simulink model "MBDMotorSystemUpd2TrqReduce95"  (R2023a)
settings: Solver=VariableStepAuto  StartTime=0.0  StopTime=0.5  RelTol=1e-3
undefined symbols (not defined in the file): CntFdqDcpMap, CntLdqDMap, CntTrqReqMap, DiscIntNeverNeededParam, Izc, Izr, MaxLmtTrq, MdlFluxMap, MdlTrqMap, Pos0
libraries: simulink x30, simulink_extras x6
(part 3 of 4)

== system MBDMotorSystemUpd2TrqReduce95/PM Controller/PM Feedback Controller/dqAxis Limitation ==
  Lmt : Inport
  Fb : Inport  Port=2
  Complex to Magnitude-Angle : ComplexToMagnitudeAngle
  Complex to Real-Imag : ComplexToRealImag
  Constant : Constant  Value=0
  Demux : Demux  Outputs=2
  Fig VltStt1 : Scope  NumInputPorts=3
  Magnitude-Angle to Complex : MagnitudeAngleToComplex
  Mux : Mux  Inputs=2
  Real-Imag to Complex : RealImagToComplex
  Saturation Dynamic : simulink/Discontinuities/Saturation Dynamic  OutMin=[]  OutMax=[]  OutDataTypeStr=Inherit: Same as second input  OutDataType=fixdt(1, 16)  OutScaling=2^-10  DoSatur=off
  Sum2 : Sum  Inputs=-+|
  Val : Outport
  Delta : Outport  Port=2
  zVal : Outport  Port=3
  wires:
  Sum2/1 -> Delta/1
  Mux/1 -> Sum2/1, Val/1
  Demux/2 -> Real-Imag to Complex/2
  Demux/1 -> Real-Imag to Complex/1
  Constant/1 -> Saturation Dynamic/3
  Complex to Real-Imag/2 -> Mux/2
  Complex to Real-Imag/1 -> Mux/1
  Complex to Magnitude-Angle/2 -> Magnitude-Angle to Complex/2
  Saturation Dynamic/1 -> Fig VltStt1/2, Magnitude-Angle to Complex/1, zVal/1
  Fb/1 -> Demux/1, Sum2/2
  Complex to Magnitude-Angle/1 -> Fig VltStt1/1, Saturation Dynamic/2
  Lmt/1 -> Fig VltStt1/3, Saturation Dynamic/1
  Magnitude-Angle to Complex/1 -> Complex to Real-Imag/1
  Real-Imag to Complex/1 -> Complex to Magnitude-Angle/1

== system MBDMotorSystemUpd2TrqReduce95/PM Controller/PWM Timer/Base Modulator ==
  Fc : Inport
  Compare To Constant : simulink/Logic and Bit Operations/Compare To Constant  relop=<=  const=-1  OutDataTypeStr=boolean
  Compare To Constant1 : simulink/Logic and Bit Operations/Compare To Constant  relop=>=  const=1  OutDataTypeStr=boolean
  Data Type Conversion : DataTypeConversion  SaturateOnIntegerOverflow=off  RndMeth=Floor
  Fcn : Fcn  Expr=2*u(1)-1
  Gain : Gain  Gain=4
  Integrator : Integrator  InitialCondition=-1
  Math Function : Math  Operator=reciprocal  SignedPower=on
  Product : Product
  S-R Flip-Flop : simulink_extras/Flip Flops/S-R Flip-Flop  initial_condition=0
  Terminator : Terminator
  sampler : Subsystem  TreatAsAtomicUnit=on  mask{lTypTrigger=1: 山}
      mask prompts: lTypTrigger "更新トリガ"
      mask TypeOptions lTypTrigger: 0: 両方 | 1: 山 | 2: 谷
      mask Callback lTypTrigger:
      | if contains(get_param(gcbh,'lTypTrigger'),'山')
      |     set_param(getSimulinkBlockHandle([gcb,'/Trigger']),'TriggerType','rising')
      | elseif contains(get_param(gcbh,'lTypTrigger'),'谷')
      |     set_param(getSimulinkBlockHandle([gcb,'/Trigger']),'TriggerType','falling')
      | else
      |     set_param(getSimulinkBlockHandle([gcb,'/Trigger']),'TriggerType','either')
      | end
  "Trigger " : Outport
  Carrier : Outport  Port=2
  Tc : Outport  Port=3
  wires:
  sampler/1(Out1) -> Gain/1, Math Function/1
  Fc/1 -> sampler/1(In1)
  Gain/1 -> Product/2
  S-R Flip-Flop/2 -> Terminator/1
  Data Type Conversion/1 -> Fcn/1, "Trigger "/1
  Product/1 -> Integrator/1
  Compare To Constant1/1 -> S-R Flip-Flop/2
  Compare To Constant/1 -> S-R Flip-Flop/1
  S-R Flip-Flop/1 -> Data Type Conversion/1
  Fcn/1 -> Product/1, sampler/Trigger
  Integrator/1 -> Compare To Constant/1, Compare To Constant1/1, Carrier/1
  Math Function/1 -> Tc/1

== system MBDMotorSystemUpd2TrqReduce95/PM Controller/PWM Timer/DeadTime Correction ==
  Tdcs : Inport
  Iuvw : Inport  Port=2
  Abs : Abs  SaturateOnIntegerOverflow=off
  Constant : Constant  Value=0
  Constant1 : Constant  Value=[0 -vThr vThr]
  Constant2 : Constant  Value=0
  Constant5 : Constant  Value=vThr
  Constant7 : Constant
  Constant8 : Constant  Value=2
  Demux : Demux  Outputs=2
  Demux1 : Demux  Outputs=3
  Detect Change : simulink/Logic and Bit Operations/Detect Change  vinit=0  OutDataTypeStr=boolean
  Gain : Gain  Gain=kCrctTd
  Gain1 : Gain  Gain=0.5
  Logical Operator : Logic  Operator=NOR  AllPortsSameDT=off  OutDataTypeStr=boolean
  Multiport Switch : MultiPortSwitch  DataPortOrder=Zero-based contiguous  zeroidx=on  SaturateOnIntegerOverflow=off  InputSameDT=off
  Multiport Switch1 : MultiPortSwitch  DataPortOrder=Zero-based contiguous  zeroidx=on  SaturateOnIntegerOverflow=off  InputSameDT=off
  Relational Operator : RelationalOperator  Operator=>  OutDataTypeStr=boolean  RndMeth=Simplest  InputSameDT=off
  Relational Operator1 : RelationalOperator  Operator=>  OutDataTypeStr=boolean  RndMeth=Simplest  InputSameDT=off
  Switch : Switch  Criteria=u2 > Threshold  SaturateOnIntegerOverflow=off  InputSameDT=off
  Switch3 : Switch  Criteria=u2 > Threshold  SaturateOnIntegerOverflow=off  InputSameDT=off
  Unit Delay : UnitDelay  SampleTime=-1  HasFrameUpgradeWarning=on
  Tdc : Outport
  wires:
  Constant5/1 -> Gain1/1
  Gain1/1 -> Relational Operator/2
  Gain/1 -> Tdc/1
  Constant2/1 -> Multiport Switch/2
  Demux/2 -> Multiport Switch/4
  Demux/1 -> Multiport Switch/3
  Constant1/1 -> Demux1/1
  Demux1/3 -> Multiport Switch1/4
  Demux1/2 -> Multiport Switch1/3
  Demux1/1 -> Multiport Switch1/2
  Constant8/1 -> Switch3/3
  Multiport Switch1/1 -> Unit Delay/1
  Tdcs/1 -> Demux/1
  Switch/1 -> Multiport Switch/1, Multiport Switch1/1
  Multiport Switch/1 -> Gain/1
  Constant7/1 -> Switch3/1
  Relational Operator1/1 -> Switch3/2
  Constant/1 -> Switch/1
  Relational Operator/1 -> Logical Operator/2
  Detect Change/1 -> Logical Operator/1
  Abs/1 -> Relational Operator/1, Detect Change/1
  Iuvw/1 -> Abs/1, Relational Operator1/1
  Switch3/1 -> Switch/3
  Logical Operator/1 -> Switch/2
  Unit Delay/1 -> Relational Operator1/2

== system MBDMotorSystemUpd2TrqReduce95/PM Controller/PWM Timer/PWM Sampler ==
  v : Inport
  Trigger : TriggerPort  VariantControl=Variant
  s : Outport  InitialOutput=[0 0 0]
  wires:
  v/1 -> s/1

== system MBDMotorSystemUpd2TrqReduce95/PM Controller/PWM Timer/Signal Offset ==
  puvw : Inport
  Constant1 : Constant  Value=2
  Constant2 : Constant  Value=0
  Constant3 : Constant  Value=-2
  Demux : Demux  Outputs=3
  Mux : Mux  Inputs=3
  Sum2 : Sum  Inputs=++|
  Sum3 : Sum  Inputs=++|
  Sum4 : Sum  Inputs=++|
  Pwm SigOuts : Outport
  wires:
  Demux/1 -> Sum2/1
  Demux/2 -> Sum3/1
  Demux/3 -> Sum4/1
  puvw/1 -> Demux/1
  Constant1/1 -> Sum2/2
  Mux/1 -> Pwm SigOuts/1
  Constant2/1 -> Sum3/2
  Sum4/1 -> Mux/3
  Constant3/1 -> Sum4/2
  Sum2/1 -> Mux/1
  Sum3/1 -> Mux/2

== system MBDMotorSystemUpd2TrqReduce95/PM Controller/Resolver Settings/Resolver Error ==
  note: 代数ループ回避
      | 誤差なので問題無と
  note: 乱数は，乱数発生器 rng での初期化が場合により必要です．
  note: 必要に応じて，追加・削除・変更して下さい．
  note: 各位置毎にテーブルでエラー設定
      | その間を線形補間
  Pos Rez. [deg.] : Inport
  Fail : Inport  Port=2
  Constant : Constant  Value=0.5
  Constant1 : Constant  Value=0
  Error Mode : Constant  Value=0
  Gain : Gain  Gain=10
  Gain1 : Gain  Gain=20
  Gain2 : Gain  Gain=2
  Manual Switch : ManualSwitch  CurrentSetting=0
  Memory : Memory  Commented=through
  Multiport Switch : MultiPortSwitch  DataPortOrder=Zero-based contiguous  Inputs=4  DataPortForDefault=Additional data port  DiagnosticForDefault=Warning  zeroidx=on  SaturateOnIntegerOverflow=off  InputSameDT=off
  Ramdom Error : Lookup_n-D  NumberOfTableDimensions=1  BreakpointsForDimension1=0:360  Table=rand(1,361)  InternalRulePriority=Speed  RndMeth=Simplest
  Sin Error : Lookup_n-D  NumberOfTableDimensions=1  BreakpointsForDimension1=0:360  Table=sind(0:360)  InternalRulePriority=Speed  RndMeth=Simplest
  Sum : Sum  Inputs=|+-
  Table Error : Lookup_n-D  NumberOfTableDimensions=1  BreakpointsForDimension1=0:30:360  BeginIndexSearchUsingPreviousIndexResult=on  Table=[10 30 -50 80 -10 50 -100 20 -50 70 -30 -80 10]  InternalRulePriority=Speed  RndMeth=Simplest
  Err. [deg.] : Outport
  wires:
  Pos Rez. [deg.]/1 -> Table Error/1, Ramdom Error/1, Sin Error/1
  Ramdom Error/1 -> Sum/1
  Sum/1 -> Gain2/1
  Constant/1 -> Sum/2
  Sin Error/1 -> Gain1/1
  Multiport Switch/1 -> Memory/1
  Manual Switch/1 -> Multiport Switch/6, Multiport Switch/1
  Gain2/1 -> Gain/1
  Memory/1 -> Err. [deg.]/1
  Gain1/1 -> Multiport Switch/5
  Gain/1 -> Multiport Switch/4
  Table Error/1 -> Multiport Switch/3
  Error Mode/1 -> Manual Switch/1
  Fail/1 -> Manual Switch/2
  Constant1/1 -> Multiport Switch/2

== system MBDMotorSystemUpd2TrqReduce95/PM Controller/Resolver Settings/Resolver Fail ==
  Pos. Mech. [deg.] : Inport
  Fail Speed [rpm] : Inport  Port=2
  Fail : Inport  Port=3
  Compare To Constant : simulink/Logic and Bit Operations/Compare To Constant  relop=<  const=0.5  OutDataTypeStr=boolean
  Gain1 : Gain  Gain=6
  Integrator1 : Integrator  ExternalReset=level  InitialConditionSource=external  InitialCondition=Pos0  WrapState=on  WrappedStateUpperValue=360  WrappedStateLowerValue=0
  NOT : Logic  Operator=NOT  IconShape=distinctive  AllPortsSameDT=off  OutDataTypeStr=boolean
  Switch : Switch  Criteria=u2 > Threshold  SaturateOnIntegerOverflow=off  InputSameDT=off
  Pos. Mech. [deg] : Outport
  wires:
  NOT/1 -> Switch/2
  Fail Speed [rpm]/1 -> Gain1/1
  Gain1/1 -> Integrator1/1
  Pos. Mech. [deg.]/1 -> Switch/3, Integrator1/3
  Compare To Constant/1 -> Integrator1/2, NOT/1
  Fail/1 -> Compare To Constant/1
  Integrator1/1 -> Switch/1
  Switch/1 -> Pos. Mech. [deg]/1

== system MBDMotorSystemUpd2TrqReduce95/Power Source/Power Source Cable Cs/Cable LR ==
  note: Inner Status
  Vin : Inport
  Vo : Inport  Port=2
  Ib0 : Inport  Port=3
  Bus Creator2 : BusCreator  Inputs=3
  Bus Creator3 : BusCreator  Inputs=3
  Constant1 : Constant  Value=0
  Constant2 : Constant  Value=0
  Divide2 : Product  Inputs=*/
  Integrator1 : Integrator  InitialConditionSource=external  LowerSaturationLimit=0
  IsRc : VariantSource  VariantControlMode=label  LabelModeActiveChoice=Off  ShowConditionOnBlock=on
  Product1 : Product
  Sum2 : Sum  Inputs=+-
  Sum6 : Sum  Inputs=+-
  vLc : Constant  Value=1e-06
  vRc : Constant  Value=0.001
  Ib : Outport
  Stt : Outport  Port=2
  wires:
  vLc/1 -> Divide2/2
  Divide2/1 -> Integrator1/1
  Integrator1/1 -> [Ib], Product1/1, Ib/1
  Vin/1 -> Sum6/1
  Vo/1 -> [Vo], Sum6/2
  vRc/1 -> Product1/2
  Ib0/1 -> Integrator1/2
  Sum6/1 -> [Vcl], Sum2/1
  Constant2/1 -> IsRc/1
  Product1/1 -> IsRc/2
  Sum2/1 -> Divide2/1
  IsRc/1 -> [Vcr], Sum2/2
  [Vcr] -> Bus Creator3/3  "Vcr"
  [Ib] -> Bus Creator2/2  "Ib"
  Constant1/1 -> Bus Creator3/2  "Icc"
  [Vcl] -> Bus Creator3/1  "Vcl"
  Bus Creator3/1 -> Bus Creator2/3  "InStt"
  Bus Creator2/1 -> Stt/1  "CblStt"
  [Vo] -> Bus Creator2/1  "Vo"

== system MBDMotorSystemUpd2TrqReduce95/Power Source/Power Source Cable Cs/Cable LRC ==
  note: Inner Status
  Vin : Inport
  Io : Inport  Port=2
  V0 : Inport  Port=3
  Bus Creator : BusCreator  Inputs=3
  Bus Creator1 : BusCreator  Inputs=3
  Constant4 : Constant  Value=0
  Divide1 : Product  Inputs=*/
  Divide2 : Product  Inputs=*/
  Integrator : Integrator  InitialConditionSource=external  LimitOutput=on  LowerSaturationLimit=0
  Integrator1 : Integrator  LowerSaturationLimit=0
  IsRc : VariantSource  VariantControlMode=label  LabelModeActiveChoice=Off  ShowConditionOnBlock=on
  Product1 : Product
  Sum1 : Sum  Inputs=+-
  Sum2 : Sum  Inputs=+-
  Sum6 : Sum  Inputs=+-
  vCc : Constant  Value=1e-06
  vLc : Constant  Value=1e-06
  vRc : Constant  Value=0.001
  Vo : Outport
  Ib : Outport  Port=2
  Stt : Outport  Port=3
  wires:
  IsRc/1 -> Sum2/2, [Vcr]
  vRc/1 -> Product1/2
  Constant4/1 -> IsRc/1
  Bus Creator1/1 -> Bus Creator/3  "InStt"
  [Vcr] -> Bus Creator1/3  "Vcr"
  [Icc] -> Bus Creator1/2  "Icc"
  [Vcl] -> Bus Creator1/1  "Vcl"
  [Ib] -> Bus Creator/2  "Ib"
  [Vo] -> Bus Creator/1  "Vo"
  Bus Creator/1 -> Stt/1  "CblStt"
  Io/1 -> Sum1/2
  Integrator/1 -> [Vo], Sum6/2, Vo/1
  Divide1/1 -> Integrator/1
  vCc/1 -> Divide1/2
  Sum1/1 -> Divide1/1, [Icc]
  Product1/1 -> IsRc/2
  Sum6/1 -> Sum2/1
  Vin/1 -> Sum6/1
  Integrator1/1 -> [Ib], Product1/1, Sum1/1, Ib/1
  Divide2/1 -> Integrator1/1
  Sum2/1 -> Divide2/1, [Vcl]
  vLc/1 -> Divide2/2
  V0/1 -> Integrator/2

== system MBDMotorSystemUpd2TrqReduce95/Power Source/Power Source Cable Cs/Cs No ESL ==
  note: Inner Status
  I Load : Inport
  Ib : Inport  Port=2
  V0in : Inport  Port=3
  Bus Creator2 : BusCreator  Inputs=3
  Bus Creator3 : BusCreator  Inputs=3
  Constant2 : Constant  Value=0
  Divide : Product  Inputs=*/
  Divide1 : Product  Inputs=*/
  Integrator : Integrator  InitialConditionSource=external  LimitOutput=on  LowerSaturationLimit=0
  IsESR : VariantSource  VariantControlMode=label  LabelModeActiveChoice=Off  ShowConditionOnBlock=on
  IsESRini : VariantSource  VariantControlMode=label  LabelModeActiveChoice=Off  ShowConditionOnBlock=on
  Product : Product
  Sum1 : Sum  Inputs=+-
  Sum2 : Sum
  Sum3 : Sum  Inputs=+-
  Sum4 : Sum  Inputs=-+
  isIR : VariantSource  VariantControlMode=label  LabelModeActiveChoice=Off  ShowConditionOnBlock=on
  vCsU : Constant  Value=Cs
  vESR : Constant  Value=ESR
  vIR : Constant  Value=IR
  Vdc : Outport
  Stt : Outport  Port=2
  wires:
  Sum4/1 -> IsESRini/1
  V0in/1 -> Sum4/2, IsESRini/2
  Integrator/1 -> [Vcs], Sum2/2, Divide1/1
  Divide/1 -> Integrator/1
  vESR/1 -> Product/1
  vCsU/1 -> Divide/2
  I Load/1 -> Sum1/2
  Ib/1 -> Sum1/1
  [Vesr] -> Sum4/1
  isIR/1 -> [Is], Divide/1
  Divide1/1 -> [Iir], Sum3/2
  Sum3/1 -> isIR/2
  Sum1/1 -> Sum3/1, isIR/1, Product/2
  vIR/1 -> Divide1/2
  IsESR/1 -> [Vesr], Sum2/1
  Sum2/1 -> [Vdc], Vdc/1
  Constant2/1 -> IsESR/2
  Product/1 -> IsESR/1
  [Vdc] -> Bus Creator2/1  "Vin"
  [Iir] -> Bus Creator3/3  "Iir"
  [Vcs] -> Bus Creator3/1  "Vcs"
  Bus Creator2/1 -> Stt/1  "CsStt"
  [Vesr] -> Bus Creator3/2  "Ver"
  [Is] -> Bus Creator2/2  "Is"
  Bus Creator3/1 -> Bus Creator2/3  "InStt"
  IsESRini/1 -> Integrator/2

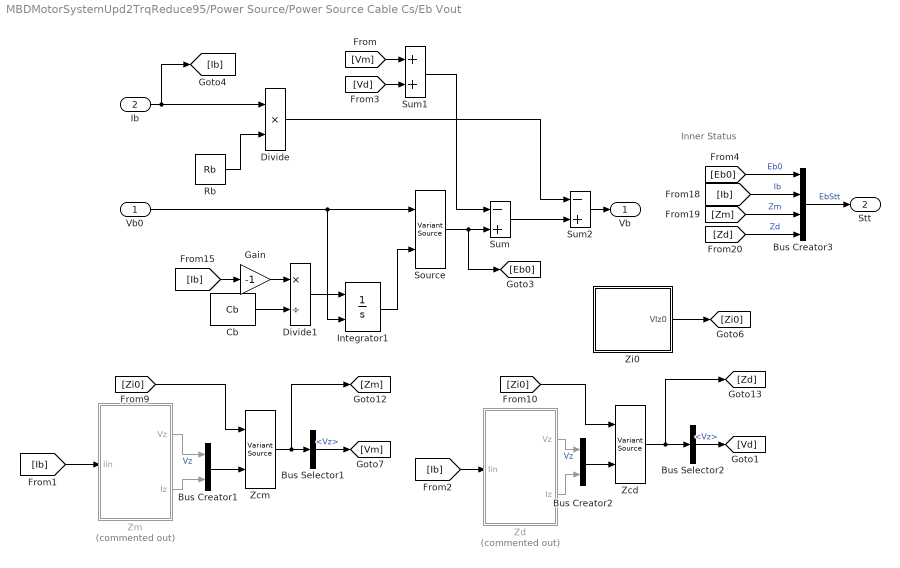
== system MBDMotorSystemUpd2TrqReduce95/Power Source/Power Source Cable Cs/Eb Vout ==
  note: Inner Status
  Vb0 : Inport
  Ib : Inport  Port=2
  Bus Creator1 : BusCreator  Inputs=2
  Bus Creator2 : BusCreator  Inputs=2
  Bus Creator3 : BusCreator  Inputs=4
  Bus Selector1 : BusSelector  OutputSignals=Vz
  Bus Selector2 : BusSelector  OutputSignals=Vz
  Cb : Constant  Value=Cb
  Divide : Product
  Divide1 : Product  Inputs=*/
  Gain : Gain  Gain=-1
  Integrator1 : Integrator  InitialConditionSource=external  LimitOutput=on  LowerSaturationLimit=0
  Rb : Constant  Value=Rb
  Source : VariantSource  VariantControlMode=label  LabelModeActiveChoice=PS  ShowConditionOnBlock=on
  Sum : Sum  Inputs=-+
  Sum1 : Sum
  Sum2 : Sum  Inputs=-+
  Zcd : VariantSource  VariantControlMode=label  LabelModeActiveChoice=Off  ShowConditionOnBlock=on
  Zcm : VariantSource  VariantControlMode=label  LabelModeActiveChoice=Off  ShowConditionOnBlock=on
  Zd : Subsystem  Commented=on  mask{Cz=Cd, Rz=Rd}
      mask prompts: Cz "内部インピーダンス容量 [C]"; Rz "内部インピーダンス抵抗 [Ω]"
      mask DialogControl ParameterGroupVar Prompt: パラメーター
  Zi0 : Subsystem
  Zm : Subsystem  Commented=on  mask{Cz=Cm, Rz=Rm}
      mask prompts: Cz "内部インピーダンス容量 [C]"; Rz "内部インピーダンス抵抗 [Ω]"
      mask DialogControl ParameterGroupVar Prompt: パラメーター
  Vb : Outport
  Stt : Outport  Port=2
  wires:
  Bus Creator3/1 -> Stt/1  "EbStt"
  [Zm] -> Bus Creator3/3  "Zm"
  [Eb0] -> Bus Creator3/1  "Eb0"
  [Ib] -> Bus Creator3/2  "Ib"
  [Zd] -> Bus Creator3/4  "Zd"
  [Zi0] -> Zcd/1
  Zcd/1 -> Bus Selector2/1, [Zd]
  Bus Selector2/1 -> [Vd]  "<Vz>"
  Zd/1(Vz) -> Bus Creator2/1  "Vz"
  Bus Creator2/1 -> Zcd/2
  Zd/2(Iz) -> Bus Creator2/2
  Zcm/1 -> Bus Selector1/1, [Zm]
  [Zi0] -> Zcm/1
  Bus Creator1/1 -> Zcm/2
  Zm/1(Vz) -> Bus Creator1/1  "Vz"
  Zm/2(Iz) -> Bus Creator1/2
  Bus Selector1/1 -> [Vm]  "<Vz>"
  Zi0/1(VIz0) -> [Zi0]
  [Ib] -> Zm/1(Iin)
  [Ib] -> Gain/1
  Rb/1 -> Divide/2
  Ib/1 -> Divide/1, [Ib]
  Sum/1 -> Sum2/2
  Gain/1 -> Divide1/1
  Divide1/1 -> Integrator1/1
  Cb/1 -> Divide1/2
  Vb0/1 -> Integrator1/2, Source/1
  Integrator1/1 -> Source/2
  Source/1 -> [Eb0], Sum/2
  [Vm] -> Sum1/1
  [Vd] -> Sum1/2
  Sum1/1 -> Sum/1
  Sum2/1 -> Vb/1
  Divide/1 -> Sum2/1
  [Ib] -> Zd/1(Iin)

== system MBDMotorSystemUpd2TrqReduce95/Power Source/Power Source Cs/Cs No ESL ==
  note: Inner Status
  I Load : Inport
  Ib : Inport  Port=2
  V0in : Inport  Port=3
  Bus Creator2 : BusCreator  Inputs=3
  Bus Creator3 : BusCreator  Inputs=3
  Constant2 : Constant  Value=0
  Divide : Product  Inputs=*/
  Divide1 : Product  Inputs=*/
  Integrator : Integrator  InitialConditionSource=external  LimitOutput=on  LowerSaturationLimit=0
  IsESR : VariantSource  VariantControlMode=label  LabelModeActiveChoice=Off  ShowConditionOnBlock=on
  IsESRini : VariantSource  VariantControlMode=label  LabelModeActiveChoice=Off  ShowConditionOnBlock=on
  Product : Product
  Sum1 : Sum  Inputs=+-
  Sum2 : Sum
  Sum3 : Sum  Inputs=+-
  Sum4 : Sum  Inputs=-+
  isIR : VariantSource  VariantControlMode=label  LabelModeActiveChoice=Off  ShowConditionOnBlock=on
  vCsU : Constant  Value=Cs
  vESR : Constant  Value=ESR
  vIR : Constant  Value=IR
  Vdc : Outport
  Stt : Outport  Port=2
  wires:
  Sum4/1 -> IsESRini/1
  V0in/1 -> Sum4/2, IsESRini/2
  Integrator/1 -> [Vcs], Sum2/2, Divide1/1
  Divide/1 -> Integrator/1
  vESR/1 -> Product/1
  vCsU/1 -> Divide/2
  I Load/1 -> Sum1/2
  Ib/1 -> Sum1/1
  [Vesr] -> Sum4/1
  isIR/1 -> [Is], Divide/1
  Divide1/1 -> [Iir], Sum3/2
  Sum3/1 -> isIR/2
  Sum1/1 -> Sum3/1, isIR/1, Product/2
  vIR/1 -> Divide1/2
  IsESR/1 -> [Vesr], Sum2/1
  Sum2/1 -> [Vdc], Vdc/1
  Constant2/1 -> IsESR/2
  Product/1 -> IsESR/1
  [Vdc] -> Bus Creator2/1  "Vin"
  [Iir] -> Bus Creator3/3  "Iir"
  [Vcs] -> Bus Creator3/1  "Vcs"
  Bus Creator2/1 -> Stt/1  "CsStt"
  [Vesr] -> Bus Creator3/2  "Ver"
  [Is] -> Bus Creator2/2  "Is"
  Bus Creator3/1 -> Bus Creator2/3  "InStt"
  IsESRini/1 -> Integrator/2

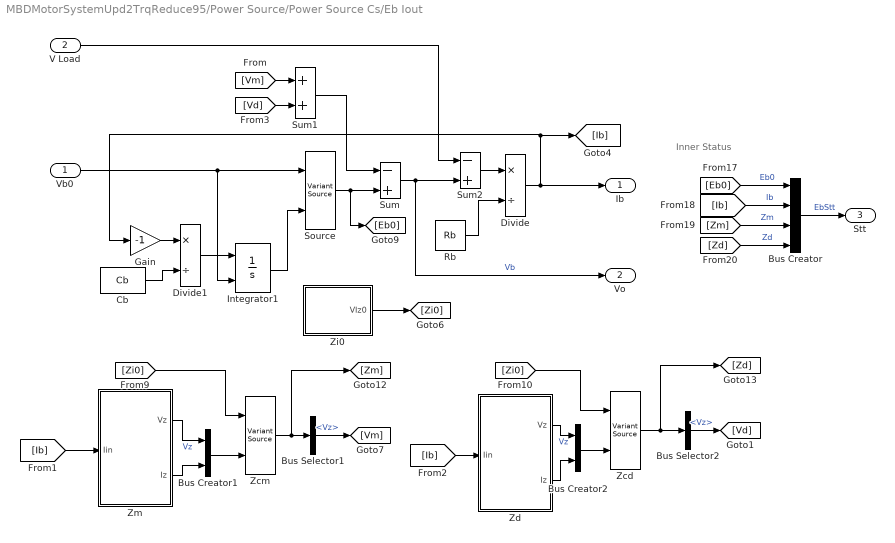
== system MBDMotorSystemUpd2TrqReduce95/Power Source/Power Source Cs/Eb Iout ==
  note: Inner Status
  Vb0 : Inport
  V Load : Inport  Port=2
  Bus Creator : BusCreator  Inputs=4
  Bus Creator1 : BusCreator  Inputs=2
  Bus Creator2 : BusCreator  Inputs=2
  Bus Selector1 : BusSelector  OutputSignals=Vz
  Bus Selector2 : BusSelector  OutputSignals=Vz
  Cb : Constant  Value=Cb
  Divide : Product  Inputs=*/
  Divide1 : Product  Inputs=*/
  Gain : Gain  Gain=-1
  Integrator1 : Integrator  InitialConditionSource=external
  Rb : Constant  Value=Rb
  Source : VariantSource  VariantControlMode=label  LabelModeActiveChoice=PS  ShowConditionOnBlock=on
  Sum : Sum  Inputs=-+
  Sum1 : Sum
  Sum2 : Sum  Inputs=-+
  Zcd : VariantSource  VariantControlMode=label  LabelModeActiveChoice=Off  ShowConditionOnBlock=on
  Zcm : VariantSource  VariantControlMode=label  LabelModeActiveChoice=Off  ShowConditionOnBlock=on
  Zd : Subsystem  mask{Cz=Cd, Rz=Rd}
      mask prompts: Cz "内部インピーダンス容量 [C]"; Rz "内部インピーダンス抵抗 [Ω]"
      mask DialogControl ParameterGroupVar Prompt: パラメーター
  Zi0 : Subsystem
  Zm : Subsystem  mask{Cz=Cm, Rz=Rm}
      mask prompts: Cz "内部インピーダンス容量 [C]"; Rz "内部インピーダンス抵抗 [Ω]"
      mask DialogControl ParameterGroupVar Prompt: パラメーター
  Ib : Outport
  Vo : Outport  Port=2
  Stt : Outport  Port=3
  wires:
  [Zi0] -> Zcm/1
  [Ib] -> Zd/1(Iin)
  [Ib] -> Zm/1(Iin)
  [Zi0] -> Zcd/1
  Zcm/1 -> Bus Selector1/1, [Zm]
  Zm/2(Iz) -> Bus Creator1/2
  Bus Selector1/1 -> [Vm]  "<Vz>"
  Zd/2(Iz) -> Bus Creator2/2
  Bus Creator2/1 -> Zcd/2
  Bus Selector2/1 -> [Vd]  "<Vz>"
  Bus Creator1/1 -> Zcm/2
  Zd/1(Vz) -> Bus Creator2/1  "Vz"
  Zcd/1 -> Bus Selector2/1, [Zd]
  Zm/1(Vz) -> Bus Creator1/1  "Vz"
  Bus Creator/1 -> Stt/1  "EbStt"
  [Zd] -> Bus Creator/4  "Zd"
  [Zm] -> Bus Creator/3  "Zm"
  [Ib] -> Bus Creator/2  "Ib"
  [Eb0] -> Bus Creator/1  "Eb0"
  Zi0/1(VIz0) -> [Zi0]
  V Load/1 -> Sum2/1
  Sum2/1 -> Divide/1
  Sum1/1 -> Sum/1
  [Vd] -> Sum1/2
  [Vm] -> Sum1/1
  Source/1 -> Sum/2, [Eb0]
  Integrator1/1 -> Source/2
  Vb0/1 -> Source/1, Integrator1/2
  Cb/1 -> Divide1/2
  Divide/1 -> Gain/1, [Ib], Ib/1
  Divide1/1 -> Integrator1/1
  Gain/1 -> Divide1/1
  Rb/1 -> Divide/2
  Sum/1 -> Vo/1, Sum2/2  "Vb"

== system MBDMotorSystemUpd2TrqReduce95/PM Controller/Modulator/Over Modulation/Ovr. Mod. ==
  PWM Mode : Inport
  Mr : Inport  Port=2
  Action Port : ActionPort  ActionPortLabel=if(u1 > 0)
  Gain : Gain  Gain=sqrt(2)/2
  Gain1 : Gain  Gain=sqrt(2)
  Merge : Merge  Inputs=3
  OvrMod. DPWM : Subsystem  TreatAsAtomicUnit=on
  OvrMod. SPWM : Subsystem  TreatAsAtomicUnit=on
  OvrMod. SVM : Subsystem  TreatAsAtomicUnit=on
  Switch Case : SwitchCase  CaseConditions={0, 1}
  Mr* : Outport
  wires:
  Switch Case/3 -> OvrMod. SPWM/Action
  OvrMod. SVM/1(Mr*) -> Merge/1
  Mr/1 -> Gain/1
  OvrMod. DPWM/1(Mr*) -> Merge/2
  Switch Case/2 -> OvrMod. DPWM/Action
  OvrMod. SPWM/1(Mr*) -> Merge/3
  PWM Mode/1 -> Switch Case/1
  Merge/1 -> Gain1/1
  Switch Case/1 -> OvrMod. SVM/Action
  Gain/1 -> OvrMod. SVM/1(Mr), OvrMod. DPWM/1(Mr), OvrMod. SPWM/1(Mr)
  Gain1/1 -> Mr*/1

== system MBDMotorSystemUpd2TrqReduce95/PM Controller/Modulator/Over Modulation/Through ==
  Mr : Inport
  Action Port : ActionPort  ActionPortLabel=else
  Mr* : Outport
  wires:
  Mr/1 -> Mr*/1

== system MBDMotorSystemUpd2TrqReduce95/PM Controller/Modulator/Vz Correction/DPWM ==
  VaReq : Inport
  MaxVa : Inport  Port=2
  Action Port : ActionPort  ActionPortLabel=case [ 1 ]:
  Abs : Abs  SaturateOnIntegerOverflow=off
  Abs1 : Abs  SaturateOnIntegerOverflow=off
  Demux3 : Demux  Outputs=3
  Demux4 : Demux  Outputs=3
  Gain : Gain  Gain=-1
  Max : MinMax  Function=max  Inputs=3  ZeroCross=off
  Max1 : MinMax  Inputs=3  ZeroCross=off
  Relational Operator3 : RelationalOperator  OutDataTypeStr=boolean  ZeroCross=off  RndMeth=Simplest  InputSameDT=off
  Sum : Sum  Inputs=-+
  Sum2 : Sum  Inputs=+-
  Switch : Switch  Criteria=u2 > Threshold  SaturateOnIntegerOverflow=off  InputSameDT=off
  Vz : Outport
  wires:
  Demux3/2 -> Max/2
  Max1/1 -> Sum/1, Abs1/1
  Demux4/3 -> Max1/3
  Demux4/2 -> Max1/2
  Demux3/3 -> Max/3
  Abs1/1 -> Relational Operator3/2
  Max/1 -> Sum2/2, Abs/1
  Abs/1 -> Relational Operator3/1
  Sum2/1 -> Switch/1
  Sum/1 -> Switch/3
  Relational Operator3/1 -> Switch/2
  VaReq/1 -> Demux3/1, Demux4/1
  Demux3/1 -> Max/1
  Demux4/1 -> Max1/1
  Switch/1 -> Vz/1
  MaxVa/1 -> [MaxVa]
  [MaxVa] -> Gain/1
  Gain/1 -> Sum/2
  [MaxVa] -> Sum2/1

== system MBDMotorSystemUpd2TrqReduce95/PM Controller/Modulator/Vz Correction/Nothing ==
  Action Port : ActionPort  ActionPortLabel=default:
  Constant : Constant  Value=0
  Vz : Outport
  wires:
  Constant/1 -> Vz/1

== system MBDMotorSystemUpd2TrqReduce95/PM Controller/Modulator/Vz Correction/SVM ==
  VaReq : Inport
  Action Port : ActionPort  ActionPortLabel=case [ 0 ]:
  Demux4 : Demux  Outputs=3
  Demux5 : Demux  Outputs=3
  Gain : Gain  Gain=-0.5
  Max : MinMax  Function=max  Inputs=3  ZeroCross=off
  Max1 : MinMax  Inputs=3  ZeroCross=off
  Mux : Mux  Inputs=2
  Sum of Elements : Sum  Inputs=+
  Vz : Outport
  wires:
  VaReq/1 -> Demux4/1, Demux5/1
  Sum of Elements/1 -> Gain/1
  Demux4/1 -> Max/1
  Demux4/3 -> Max/3
  Mux/1 -> Sum of Elements/1
  Gain/1 -> Vz/1
  Max1/1 -> Mux/2
  Demux5/1 -> Max1/1
  Demux5/3 -> Max1/3
  Max/1 -> Mux/1
  Demux5/2 -> Max1/2
  Demux4/2 -> Max/2

== system MBDMotorSystemUpd2TrqReduce95/PM Controller/PWM Timer/Base Modulator/sampler ==
  In1 : Inport
  Trigger : TriggerPort  VariantControl=Variant  InitialTriggerSignalState=zero
  Out1 : Outport
  wires:
  In1/1 -> Out1/1

== system MBDMotorSystemUpd2TrqReduce95/Power Source/Power Source Cable Cs/Eb Vout/Zd ==
  Iin : Inport
  Cz : Constant  Value=Cz
  Divide : Product  Inputs=*/
  Divide1 : Product  Inputs=*/
  Integrator : Integrator  InitialConditionSource=external
  Istt : BusCreator  Inputs=Izr,Izc
  Product : Product
  Rz : Constant  Value=Rz
  Sum : Sum  Inputs=-+
  Vz : Outport
  Iz : Outport  Port=2
  wires:
  Integrator/1 -> Divide1/1, Vz/1  "Vz"
  Istt/1 -> Iz/1  "Iz"
  Divide/1 -> Integrator/1
  Rz/1 -> Product/1, Divide1/2
  Iin/1 -> Sum/2, Product/2
  Sum/1 -> Istt/2, Divide/1  "Izc"
  Divide1/1 -> Istt/1, Sum/1  "Izr"
  Product/1 -> Integrator/2
  Cz/1 -> Divide/2

== system MBDMotorSystemUpd2TrqReduce95/Power Source/Power Source Cable Cs/Eb Vout/Zi0 ==
  Constant2 : Constant  Value=NaN
  Constant3 : Constant  Value=NaN
  Constant4 : Constant  Value=0
  Iz : BusCreator  Inputs=Izr,Izc
  VIz : BusCreator  Inputs=2
  VIz0 : Outport
  wires:
  Constant2/1 -> Iz/2  "Izc"
  Iz/1 -> VIz/2  "Iz"
  VIz/1 -> VIz0/1  "VIz"
  Constant3/1 -> Iz/1  "Izr"
  Constant4/1 -> VIz/1  "Vz"

== system MBDMotorSystemUpd2TrqReduce95/Power Source/Power Source Cable Cs/Eb Vout/Zm ==
  Iin : Inport
  Cz : Constant  Value=Cz
  Divide : Product  Inputs=*/
  Divide1 : Product  Inputs=*/
  Integrator : Integrator  InitialConditionSource=external
  Istt : BusCreator  Inputs=Izr,Izc
  Product : Product
  Rz : Constant  Value=Rz
  Sum : Sum  Inputs=-+
  Vz : Outport
  Iz : Outport  Port=2
  wires:
  Divide/1 -> Integrator/1
  Divide1/1 -> Istt/1, Sum/1  "Izr"
  Sum/1 -> Istt/2, Divide/1  "Izc"
  Cz/1 -> Divide/2
  Istt/1 -> Iz/1  "Iz"
  Product/1 -> Integrator/2
  Iin/1 -> Sum/2, Product/2
  Rz/1 -> Product/1, Divide1/2
  Integrator/1 -> Divide1/1, Vz/1  "Vz"

== system MBDMotorSystemUpd2TrqReduce95/Power Source/Power Source Cs/Eb Iout/Zd ==
  Iin : Inport
  Cz : Constant  Value=Cz
  Divide : Product  Inputs=*/
  Divide1 : Product  Inputs=*/
  Integrator : Integrator  InitialConditionSource=external
  Istt : BusCreator  Inputs=Izr,Izc
  Product : Product
  Rz : Constant  Value=Rz
  Sum : Sum  Inputs=-+
  Vz : Outport
  Iz : Outport  Port=2
  wires:
  Integrator/1 -> Divide1/1, Vz/1  "Vz"
  Istt/1 -> Iz/1  "Iz"
  Divide/1 -> Integrator/1
  Rz/1 -> Product/1, Divide1/2
  Iin/1 -> Sum/2, Product/2
  Sum/1 -> Istt/2, Divide/1  "Izc"
  Divide1/1 -> Istt/1, Sum/1  "Izr"
  Product/1 -> Integrator/2
  Cz/1 -> Divide/2

== system MBDMotorSystemUpd2TrqReduce95/Power Source/Power Source Cs/Eb Iout/Zi0 ==
  Constant1 : Constant  Value=0
  Constant2 : Constant  Value=NaN
  Constant3 : Constant  Value=NaN
  Constant4 : Constant  Value=0
  Iz : BusCreator  Inputs=Izr,Izc
  VIz : BusCreator  Inputs=3
  VIz0 : Outport
  wires:
  Constant1/1 -> VIz/3  "Vz0"
  Constant2/1 -> Iz/2  "Izc"
  Iz/1 -> VIz/2  "Iz"
  VIz/1 -> VIz0/1  "VIz"
  Constant3/1 -> Iz/1  "Izr"
  Constant4/1 -> VIz/1  "Vz"

== system MBDMotorSystemUpd2TrqReduce95/Power Source/Power Source Cs/Eb Iout/Zm ==
  Iin : Inport
  Cz : Constant  Value=Cz
  Divide : Product  Inputs=*/
  Divide1 : Product  Inputs=*/
  Integrator : Integrator  InitialConditionSource=external
  Istt : BusCreator  Inputs=Izr,Izc
  Product : Product
  Rz : Constant  Value=Rz
  Sum : Sum  Inputs=-+
  Vz : Outport
  Iz : Outport  Port=2
  wires:
  Divide/1 -> Integrator/1
  Divide1/1 -> Istt/1, Sum/1  "Izr"
  Sum/1 -> Istt/2, Divide/1  "Izc"
  Cz/1 -> Divide/2
  Istt/1 -> Iz/1  "Iz"
  Product/1 -> Integrator/2
  Iin/1 -> Sum/2, Product/2
  Rz/1 -> Product/1, Divide1/2
  Integrator/1 -> Divide1/1, Vz/1  "Vz"

== system MBDMotorSystemUpd2TrqReduce95/PM Controller/Modulator/Over Modulation/Ovr. Mod./OvrMod. DPWM ==
  Mr : Inport
  Action Port : ActionPort  ActionPortLabel=case [ 1 ]:
  Compare To Constant : simulink/Logic and Bit Operations/Compare To Constant  relop=>  const=1/sqrt(2)  OutDataTypeStr=boolean
  Ovr DPWM : Lookup_n-D  NumberOfTableDimensions=1  BreakpointsForDimension1=[0.7, 0.7001, 0.7002, 0.7003, 0.7004, 0.7005, 0.7006, 0.7007, 0.7008, 0.7009, 0.701, 0.7011, 0.7012, 0.7013, 0.7014, 0.7015, 0.7016, 0.7017, 0.7018, 0.7019, 0.702, 0.7021, 0.7022, 0.7023, 0.7024, 0.7025, 0.7026, 0.7027, 0.7028, 0.7029, 0.703, 0.7031, 0.7032, 0.7033, 0.7034, 0.7035, 0.7036, 0.7037, 0.7038, 0.7039, 0.704, 0.7041, 0.7042, 0.7043, 0.7044, 0.7045, 0.7046, 0.7047, 0.7048, 0.7049, 0.705, 0.7051, 0.7052, 0.7053, 0.7054, 0.7055, 0.7056, 0.7057, 0.7058, 0.7059, 0.706, 0.7061, 0.7062, 0.7063, 0.7064, 0.7065, 0.7066, 0.7067, 0.7068, 0.7069, 0.707, 0.7071, 0.7072, 0.7073, 0.7074, 0.7075, 0.7076, 0.7077, 0.7078, 0.7079, 0.708, 0.7081, 0.7082, 0.7083, 0.7084, 0.7085, 0.7086, 0.7087, 0.7088, 0.7089, 0.709, 0.7091, 0.7092, 0.7093, 0.7094, 0.7095, 0.7096, 0.7097, 0.7098, 0.7099, 0.71, 0.7101, 0.7102, 0.7103, 0.7104, 0.7105, 0.7106, 0.7107, 0.7108, 0.7109, 0.711, 0.7111, 0.7112, 0.7113, 0.7114, 0.7115, 0.7116, 0.7117, 0.7118, 0.7119, 0.712, 0.7121, 0.7122, 0.7123, 0.7124, 0.7125, 0.7126, 0.7127, 0.7128, 0.7129, 0.713, 0.7131, 0.7132, 0.7133, 0.7134, 0.7135, 0.7136, 0.7137, 0.7138, 0.7139, 0.714, 0.7141, 0.7142, 0.7143, 0.7144, 0.7145, 0.7146, 0.7147, 0.7148, 0.7149, 0.715, 0.7151, 0.7152, 0.7153, 0.7154, 0.7155, 0.7156, 0.7157, 0.7158, 0.7159, 0.716, 0.7161, 0.7162, 0.7163, 0.7164, 0.7165, 0.7166, 0.7167, 0.7168, 0.7169, 0.717, 0.7171, 0.7172, 0.7173, 0.7174, 0.7175, 0.7176, 0.7177, 0.7178, 0.7179, 0.718, 0.7181, 0.7182, 0.7183, 0.7184, 0.7185, 0.7186, 0.7187, 0.7188, 0.7189, 0.719, 0.7191, 0.7192, 0.7193, 0.7194, 0.7195, 0.7196, 0.7197, 0.7198, 0.7199, 0.72, 0.7201, 0.7202, 0.7203, 0.7204, 0.7205, 0.7206, 0.7207, 0.7208, 0.7209, 0.721, 0.7211, 0.7212, 0.7213, 0.7214, 0.7215, 0.7216, 0.7217, 0.7218, 0.7219, 0.722, 0.7221, 0.7222, 0.7223, 0.7224, 0.7225, 0.7226, 0.7227, 0.7228, 0.7229, 0.723, 0.7231, 0.7232, 0.7233, 0.7234, 0.7235, 0.7236, 0.7237, 0.7238, 0.7239, 0.724, 0.7241, 0.7242, 0.7243, 0.7244, 0.7245, 0.7246, 0.7247, 0.7248, 0.7249, 0.725, 0.7251, 0.7252, 0.7253, 0.7254, 0.7255, 0.7256, 0.7257, 0.7258, 0.7259, 0.726, 0.7261, 0.7262, 0.7263, 0.7264, 0.7265, 0.7266, 0.7267, 0.7268, 0.7269, 0.727, 0.7271, 0.7272, 0.7273, 0.7274, 0.7275, 0.7276, 0.7277, 0.7278, 0.7279, 0.728, 0.7281, 0.7282, 0.7283, 0.7284, 0.7285, 0.7286, 0.7287, 0.7288, 0.7289, 0.729, 0.7291, 0.7292, 0.7293, 0.7294, 0.7295, 0.7296, 0.7297, 0.7298, 0.7299, 0.73, 0.7301, 0.7302, 0.7303, 0.7304, 0.7305, 0.7306, 0.7307, 0.7308, 0.7309, 0.731, 0.7311, 0.7312, 0.7313, 0.7314, 0.7315, 0.7316, 0.7317, 0.7318, 0.7319, 0.732, 0.7321, 0.7322, 0.7323, 0.7324, 0.7325, 0.7326, 0.7327, 0.7328, 0.7329, 0.733, 0.7331, 0.7332, 0.7333, 0.7334, 0.7335, 0.7336, 0.7337, 0.7338, 0.7339, 0.734, 0.7341, 0.7342, 0.7343, 0.7344, 0.7345, 0.7346, 0.7347, 0.7348, 0.7349, 0.735, 0.7351, 0.7352, 0.7353, 0.7354, 0.7355, 0.7356, 0.7357, 0.7358, 0.7359, 0.736, 0.7361, 0.7362, 0.7363, 0.7364, 0.7365, 0.7366, 0.7367, 0.7368, 0.7369, 0.737, 0.7371, 0.7372, 0.7373, 0.7374, 0.7375, 0.7376, 0.7377, 0.7378, 0.7379, 0.738, 0.7381, 0.7382, 0.7383, 0.7384, 0.7385, 0.7386, 0.7387, 0.7388, 0.7389, 0.739, 0.7391, 0.7392, 0.7393, 0.7394, 0.7395, 0.7396, 0.7397, 0.7398, 0.7399, 0.74, 0.7401, 0.7402, 0.7403, 0.7404, 0.7405, 0.7406, 0.7407, 0.7408, 0.7409, 0.741, 0.7411, 0.7412, 0.7413, 0.7414, 0.7415, 0.7416, 0.7417, 0.7418, 0.7419, 0.742, 0.7421, 0.7422, 0.7423, 0.7424, 0.7425, 0.7426, 0.7427, 0.7428, 0.7429, 0.743, 0.7431, 0.7432, 0.7433, 0.7434, 0.7435, 0.7436, 0.7437, 0.7438, 0.7439, 0.744, 0.7441, 0.7442, 0.7443, 0.7444, 0.7445, 0.7446, 0.7447, 0.7448, 0.7449, 0.745, 0.7451, 0.7452, 0.7453, 0.7454, 0.7455, 0.7456, 0.7457, 0.7458, 0.7459, 0.746, 0.7461, 0.7462, 0.7463, 0.7464, 0.7465, 0.7466, 0.7467, 0.7468, 0.7469, 0.747, 0.7471, 0.7472, 0.7473, 0.7474, 0.7475, 0.7476, 0.7477, 0.7478, 0.7479, 0.748, 0.7481, 0.7482, 0.7483, 0.7484, 0.7485, 0.7486, 0.7487, 0.7488, 0.7489, 0.749, 0.7491, 0.7492, 0.7493, 0.7494, 0.7495, 0.7496, 0.7497, 0.7498, 0.7499, 0.75, 0.7501, 0.7502, 0.7503, 0.7504, 0.7505, 0.7506, ...(+2240 chars)]  IndexSearchMethod=Evenly spaced points  Table=[0.7, 0.7001, 0.7002, 0.7003, 0.7004, 0.7005, 0.7006, 0.7007, 0.7008, 0.7009, 0.701, 0.7011, 0.7012, 0.7013, 0.7014, 0.7015, 0.7016, 0.7017, 0.7018, 0.7019, 0.702, 0.7021, 0.7022, 0.7023, 0.7024, 0.7025, 0.7026, 0.7027, 0.7028, 0.7029, 0.703, 0.7031, 0.7032, 0.7033, 0.7034, 0.7035, 0.7036, 0.7037, 0.7038, 0.7039, 0.704, 0.7041, 0.7042, 0.7043, 0.7044, 0.7045, 0.7046, 0.7047, 0.7048, 0.7049, 0.705, 0.7051, 0.7052, 0.7053, 0.7054, 0.7055, 0.7056, 0.7057, 0.7058, 0.7059, 0.706, 0.7061, 0.706199, 0.706298, 0.706397, 0.706496, 0.706596, 0.706696, 0.706796, 0.706898, 0.707, 0.707103, 0.707207, 0.707311, 0.707416, 0.707522, 0.707629, 0.707736, 0.707844, 0.707952, 0.708062, 0.708173, 0.708284, 0.708397, 0.70851, 0.708624, 0.708739, 0.708854, 0.708969, 0.709085, 0.709201, 0.709318, 0.709436, 0.709554, 0.709673, 0.709792, 0.709911, 0.710031, 0.710151, 0.710272, 0.710394, 0.710516, 0.710638, 0.710761, 0.710884, 0.711008, 0.711132, 0.711257, 0.711382, 0.711508, 0.711634, 0.71176, 0.711887, 0.712014, 0.712142, 0.71227, 0.712399, 0.712528, 0.712657, 0.712787, 0.712917, 0.713048, 0.713179, 0.713311, 0.713443, 0.713575, 0.713708, 0.713841, 0.713975, 0.714109, 0.714243, 0.714378, 0.714513, 0.714649, 0.714785, 0.714922, 0.715059, 0.715196, 0.715334, 0.715472, 0.71561, 0.715749, 0.715889, 0.716029, 0.716169, 0.716309, 0.71645, 0.716592, 0.716734, 0.716876, 0.717018, 0.717161, 0.717305, 0.717449, 0.717593, 0.717738, 0.717883, 0.718028, 0.718174, 0.71832, 0.718467, 0.718614, 0.718762, 0.71891, 0.719058, 0.719207, 0.719356, 0.719505, 0.719655, 0.719806, 0.719956, 0.720107, 0.720259, 0.720411, 0.720563, 0.720716, 0.720869, 0.721023, 0.721177, 0.721332, 0.721486, 0.721642, 0.721797, 0.721954, 0.72211, 0.722267, 0.722424, 0.722582, 0.72274, 0.722899, 0.723058, 0.723217, 0.723377, 0.723537, 0.723698, 0.723859, 0.724021, 0.724183, 0.724345, 0.724508, 0.724671, 0.724835, 0.724999, 0.725163, 0.725328, 0.725494, 0.72566, 0.725826, 0.725992, 0.72616, 0.726327, 0.726495, 0.726663, 0.726832, 0.727001, 0.727171, 0.727341, 0.727512, 0.727683, 0.727854, 0.728026, 0.728199, 0.728371, 0.728545, 0.728718, 0.728892, 0.729067, 0.729242, 0.729417, 0.729593, 0.72977, 0.729946, 0.730124, 0.730301, 0.73048, 0.730658, 0.730837, 0.731017, 0.731197, 0.731377, 0.731558, 0.73174, 0.731921, 0.732104, 0.732287, 0.73247, 0.732654, 0.732838, 0.733022, 0.733208, 0.733393, 0.733579, 0.733766, 0.733953, 0.73414, 0.734328, 0.734517, 0.734706, 0.734895, 0.735085, 0.735276, 0.735466, 0.735658, 0.73585, 0.736042, 0.736235, 0.736428, 0.736622, 0.736817, 0.737011, 0.737207, 0.737403, 0.737599, 0.737796, 0.737993, 0.738191, 0.73839, 0.738588, 0.738788, 0.738988, 0.739188, 0.739389, 0.739591, 0.739793, 0.739995, 0.740198, 0.740402, 0.740606, 0.74081, 0.741016, 0.741221, 0.741428, 0.741634, 0.741842, 0.742049, 0.742258, 0.742467, 0.742676, 0.742886, 0.743097, 0.743308, 0.743519, 0.743732, 0.743944, 0.744158, 0.744372, 0.744586, 0.744801, 0.745017, 0.745233, 0.745449, 0.745667, 0.745884, 0.746103, 0.746322, 0.746541, 0.746762, 0.746982, 0.747204, 0.747425, 0.747648, 0.747871, 0.748095, 0.748319, 0.748544, 0.748769, 0.748995, 0.749222, 0.749449, 0.749677, 0.749905, 0.750135, 0.750364, 0.750595, 0.750825, 0.751057, 0.751289, 0.751522, 0.751755, 0.751989, 0.752224, 0.752459, 0.752695, 0.752932, 0.753169, 0.753407, 0.753646, 0.753885, 0.754125, 0.754365, 0.754606, 0.754848, 0.755091, 0.755334, 0.755577, 0.755822, 0.756067, 0.756313, 0.756559, 0.756806, 0.757054, 0.757303, 0.757552, 0.757802, 0.758053, 0.758304, 0.758556, 0.758809, 0.759062, 0.759316, 0.759571, 0.759826, 0.760083, 0.76034, 0.760597, 0.760856, 0.761115, 0.761375, 0.761635, 0.761897, 0.762159, 0.762422, 0.762685, 0.76295, 0.763215, 0.763481, 0.763747, 0.764015, 0.764283, 0.764552, 0.764821, 0.765092, 0.765363, 0.765635, 0.765908, 0.766181, 0.766456, 0.766731, 0.767007, 0.767284, 0.767562, 0.76784, 0.768119, 0.768399, 0.76868, 0.768962, 0.769244, 0.769528, 0.769812, 0.770097, 0.770383, 0.77067, 0.770957, 0.771246, 0.771535, 0.771825 ...(+3671 chars)]  ExtrapMethod=Clip  UseLastTableValue=on  ApplyFullPrecisionForLinearInterpolation=on  InternalRulePriority=Speed  RndMeth=Simplest
  Switch : Switch  Criteria=u2 > Threshold  SaturateOnIntegerOverflow=off  InputSameDT=off
  Mr* : Outport
  wires:
  Ovr DPWM/1 -> Switch/1
  Compare To Constant/1 -> Switch/2
  Mr/1 -> Ovr DPWM/1, Compare To Constant/1, Switch/3  "Normal"
  Switch/1 -> Mr*/1
